simulink model "htx_ekf_base"  (R2024b)
settings: Solver=FixedStepAuto  StartTime=0.0  StopTime=10.0  RelTol=1e-3
undefined symbols (not defined in the file): chi, GR, params, rpm2rad_s, segment_data
libraries: simulink_extras x4, matrix_library x1
settings Model: Creator=lukec  LastModifiedBy=lukec
settings OptimizationCC: DefaultParameterBehavior=Inlined  EnhancedBackFolding=on  PassReuseOutputArgsAs=Individual arguments  ZeroExternalMemoryAtStartup=off  ZeroInternalMemoryAtStartup=off  OptimizeBlockOrder=speed  DifferentSizesBufferReuse=on  OptimizationCustomize=off  EfficientTunableParamExpr=on
settings DebuggingCC: ParameterTunabilityLossMsg=error
settings HardwareCC: ProdBitPerPointer=32  ProdBitPerSizeT=32  ProdBitPerPtrDiffT=32  ProdLargestAtomicInteger=Long  ProdLargestAtomicFloat=Double  ProdWordSize=32  ProdHWDeviceType=ARM Compatible->ARM Cortex-M
settings SFSimCC: MATLABDynamicMemAlloc=off
settings RTWCC: Description=Embedded Coder  SystemTargetFile=ert.tlc  GenCodeOnly=on  PackageGeneratedCodeAndArtifacts=on  TemplateMakefile=ert_default_tmf  Toolchain=CMake  TargetLang=C++
settings CodeAppCC: ForceParamTrailComments=on  IgnoreCustomStorageClasses=off  MaxIdLength=255  OperatorAnnotations=on  SimulinkDataObjDesc=on  SFDataObjDesc=on  InsertBlockDesc=on
settings ERTTargetCC: TargetLangStandard=C++17 (ISO)  CodeInterfacePackaging=C++ class  RootIOFormat=Structure reference  ERTCustomFileTemplate=example_file_process.tlc  ArrayContainerType=std::array

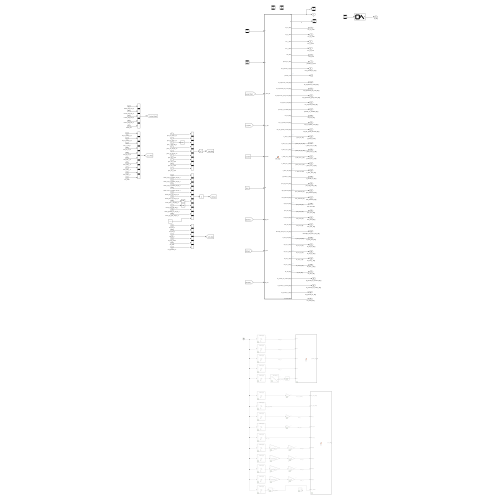
[thumbnail: Simulink's stored preview of the top-level diagram]
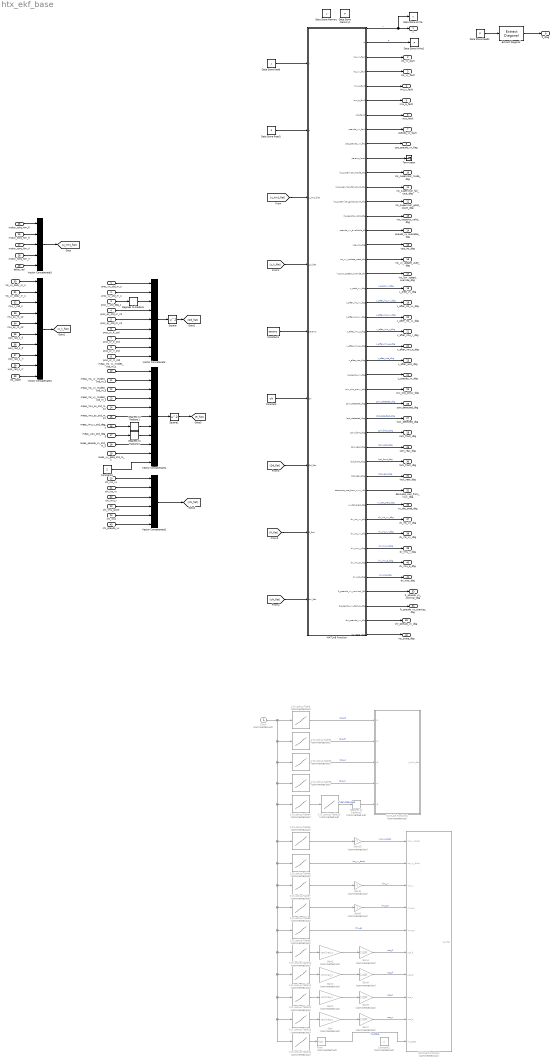
== system htx_ekf_base ==
  proc_vx_std_m_s : Inport
  proc_vy_std_m_s : Inport  Port=2
  proc_r_std_deg_s : Inport  Port=3
  proc_ax_std_m_s2 : Inport  Port=4
  proc_ay_std_m_s2 : Inport  Port=5
  proc_sr_fl_std : Inport  Port=6
  proc_sr_fr_std : Inport  Port=7
  proc_sr_rl_std : Inport  Port=8
  proc_sr_rr_std : Inport  Port=9
  meas_ins_vx_mode1_std_m_s : Inport  Port=10
  meas_ins_vy_mode1_std_m_s : Inport  Port=11
  meas_ins_vx_mode2_std_m_s : Inport  Port=12
  meas_ins_vy_mode2_std_m_s : Inport  Port=13
  meas_imu_ax_std_m_s2 : Inport  Port=14
  meas_imu_ay_std_m_s2 : Inport  Port=15
  meas_imu_r_std_deg_s : Inport  Port=16
  meas_wss_std_deg_s : Inport  Port=17
  meas_pseudo_vx_std_m_s : Inport  Port=18
  meas_vy_gate_std_m_s : Inport  Port=19
  chi_ins_vx : Inport  Port=20
  chi_ins_vy : Inport  Port=21
  chi_imu_r : Inport  Port=22
  chi_imu_accel : Inport  Port=23
  chi_wss : Inport  Port=24
  motor_torq_Nm_fl : Inport  Port=25
  motor_torq_Nm_fr : Inport  Port=26
  motor_torq_Nm_rl : Inport  Port=27
  motor_torq_Nm_rr : Inport  Port=28
  delta_rad : Inport  Port=29
  ins_vx_body_m_s : Inport  Port=30
  ins_vy_body_m_s : Inport  Port=31
  imu_r_rad_s : Inport  Port=32
  imu_ax_m_s2 : Inport  Port=33
  imu_ay_m_s2 : Inport  Port=34
  wss_rad_s_fl : Inport  Port=35
  wss_rad_s_fr : Inport  Port=36
  wss_rad_s_rl : Inport  Port=37
  wss_rad_s_rr : Inport  Port=38
  ins_state : Inport  Port=39
  chi_pseudo_vx : Inport  Port=40
  1-D Lookup Table : Lookup_n-D  Commented=on  NumberOfTableDimensions=1  BreakpointsForDimension1=segment_data.globalTime  Table=segment_data.inv1_dynamics.actual_torque_nm  ExtrapMethod=Clip  InternalRulePriority=Speed  RndMeth=Simplest
  1-D Lookup Table1 : Lookup_n-D  Commented=on  NumberOfTableDimensions=1  BreakpointsForDimension1=segment_data.globalTime  Table=segment_data.inv2_dynamics.actual_torque_nm  ExtrapMethod=Clip  InternalRulePriority=Speed  RndMeth=Simplest
  1-D Lookup Table10 : Lookup_n-D  Commented=on  NumberOfTableDimensions=1  BreakpointsForDimension1=segment_data.globalTime  Table=segment_data.inv1_dynamics.actual_speed_rpm  ExtrapMethod=Clip  InternalRulePriority=Speed  RndMeth=Simplest
  1-D Lookup Table11 : Lookup_n-D  Commented=on  NumberOfTableDimensions=1  BreakpointsForDimension1=segment_data.globalTime  Table=segment_data.inv2_dynamics.actual_speed_rpm  ExtrapMethod=Clip  InternalRulePriority=Speed  RndMeth=Simplest
  1-D Lookup Table12 : Lookup_n-D  Commented=on  NumberOfTableDimensions=1  BreakpointsForDimension1=segment_data.globalTime  Table=segment_data.inv3_dynamics.actual_speed_rpm  ExtrapMethod=Clip  InternalRulePriority=Speed  RndMeth=Simplest
  1-D Lookup Table13 : Lookup_n-D  Commented=on  NumberOfTableDimensions=1  BreakpointsForDimension1=segment_data.globalTime  Table=segment_data.inv4_dynamics.actual_speed_rpm  ExtrapMethod=Clip  InternalRulePriority=Speed  RndMeth=Simplest
  1-D Lookup Table14 : Lookup_n-D  Commented=on  NumberOfTableDimensions=1  BreakpointsForDimension1=segment_data.globalTime  Table=segment_data.VNData.status.ins_mode_int  ExtrapMethod=Clip  InternalRulePriority=Speed  RndMeth=Simplest
  1-D Lookup Table15 : Lookup_n-D  Commented=on  NumberOfTableDimensions=1  BreakpointsForDimension1=[1060 3010]  Table=[23 -23]  ExtrapMethod=Clip  InternalRulePriority=Speed  RndMeth=Simplest
  1-D Lookup Table2 : Lookup_n-D  Commented=on  NumberOfTableDimensions=1  BreakpointsForDimension1=segment_data.globalTime  Table=segment_data.inv3_dynamics.actual_torque_nm  ExtrapMethod=Clip  InternalRulePriority=Speed  RndMeth=Simplest
  1-D Lookup Table3 : Lookup_n-D  Commented=on  NumberOfTableDimensions=1  BreakpointsForDimension1=segment_data.globalTime  Table=segment_data.inv4_dynamics.actual_torque_nm  ExtrapMethod=Clip  InternalRulePriority=Speed  RndMeth=Simplest
  1-D Lookup Table4 : Lookup_n-D  Commented=on  NumberOfTableDimensions=1  BreakpointsForDimension1=segment_data.globalTime  Table=segment_data.steering_data.steering_analog_raw  ExtrapMethod=Clip  InternalRulePriority=Speed  RndMeth=Simplest
  1-D Lookup Table5 : Lookup_n-D  Commented=on  NumberOfTableDimensions=1  BreakpointsForDimension1=segment_data.globalTime  Table=segment_data.VNData.vn_vel_m_s.x  ExtrapMethod=Clip  InternalRulePriority=Speed  RndMeth=Simplest
  1-D Lookup Table6 : Lookup_n-D  Commented=on  NumberOfTableDimensions=1  BreakpointsForDimension1=segment_data.globalTime  Table=segment_data.VNData.vn_vel_m_s.y  ExtrapMethod=Clip  InternalRulePriority=Speed  RndMeth=Simplest
  1-D Lookup Table7 : Lookup_n-D  Commented=on  NumberOfTableDimensions=1  BreakpointsForDimension1=segment_data.globalTime  Table=segment_data.VNData.vn_angular_rate_rad_s.z  ExtrapMethod=Clip  InternalRulePriority=Speed  RndMeth=Simplest
  1-D Lookup Table8 : Lookup_n-D  Commented=on  NumberOfTableDimensions=1  BreakpointsForDimension1=segment_data.globalTime  Table=segment_data.VNData.vn_linear_accel_m_ss.x  ExtrapMethod=Clip  InternalRulePriority=Speed  RndMeth=Simplest
  1-D Lookup Table9 : Lookup_n-D  Commented=on  NumberOfTableDimensions=1  BreakpointsForDimension1=segment_data.globalTime  Table=segment_data.VNData.vn_linear_accel_m_ss.y  ExtrapMethod=Clip  InternalRulePriority=Speed  RndMeth=Simplest
  Clock : Clock  Commented=on
  Constant : Constant  Value=chi  OutDataTypeStr=Bus: chi_bus
  Constant1 : Constant  Value=params  OutDataTypeStr=Bus: params_bus
  Constant2 : Constant  Commented=on  Value=0
  Constant3 : Constant  Value=2
  Data Store Memory : DataStoreMemory  DataStoreName=x  WriteAfterWriteMsg=warning  InitialValue=x0  ShowAdditionalParam=off
  Data Store Memory1 : DataStoreMemory  DataStoreName=P  WriteAfterWriteMsg=warning  InitialValue=P0  ShowAdditionalParam=off
  Data Store Read : DataStoreRead  DataStoreName=x  IndexOptions=Index vector (dialog)  Indices=1  OutputSizes=1
  Data Store Read1 : DataStoreRead  DataStoreName=P  IndexOptions=Index vector (dialog)  Indices=1  OutputSizes=1
  Data Store Read2 : DataStoreRead  DataStoreName=P  IndexOptions=Index vector (dialog)  Indices=1  OutputSizes=1
  Data Store Write : DataStoreWrite  DataStoreName=x  IndexOptions=Index vector (dialog)  Indices=1  OutputSizes=1
  Data Store Write1 : DataStoreWrite  DataStoreName=P  IndexOptions=Index vector (dialog)  Indices=1  OutputSizes=1
  Degrees to Radians : simulink_extras/Transformations/Degrees to Radians
  Degrees to Radians1 : simulink_extras/Transformations/Degrees to Radians
  Degrees to Radians2 : simulink_extras/Transformations/Degrees to Radians
  Degrees to Radians3 : simulink_extras/Transformations/Degrees to Radians  Commented=on
  Extract Diagonal : matrix_library/Extract Diagonal
      settings: LibrarySourceBlock=|
      | simulink/Matrix
      | Operations/Extract Diagonal
  Floor : Rounding  Commented=on
  Gain{,1..3} (4 alike) : Gain  Commented=on  Gain=rpm2rad_s
  Gain10 : Gain  Commented=on  Gain=-1
  Gain{4..7} (4 alike) : Gain  Commented=on  Gain=1/GR
  Gain8 : Gain  Commented=on  Gain=-1
  Gain9 : Gain  Commented=on  Gain=-1
  MATLAB Function : MATLAB Function  TreatAsAtomicUnit=on
  MATLAB Function1 : MATLAB Function  Commented=on  TreatAsAtomicUnit=on
  MATLAB Function2 : MATLAB Function  Commented=on  TreatAsAtomicUnit=on
  Square : Math  Operator=square
  Square1 : Math  Operator=square
  Terminator : Terminator
  Vector Concatenate : Concatenate  NumInputs=9
  Vector Concatenate1 : Concatenate  NumInputs=11
  Vector Concatenate2 : Concatenate  NumInputs=6
  Vector Concatenate3 : Concatenate  NumInputs=5
  Vector Concatenate4 : Concatenate  NumInputs=10
  x : Outport
  ins_vx_fault : Outport  Port=2
  ins_vy_fault : Outport  Port=3
  imu_r_fault : Outport  Port=4
  imu_a_fault : Outport  Port=5
  wss_fault : Outport  Port=6
  pseudo_vx_fault : Outport  Port=7
  use_pseudo_vx_flag : Outport  Port=8
  P_diag : Outport  Port=9
  ins_supervisor_mode_dbg : Outport  Port=10
  ins_supervisor_fail_cout_dbg : Outport  Port=11
  ins_supervisor_good_count_dbg : Outport  Port=12
  ins_resports_valid_dbg : Outport  Port=13
  pseudo_vx_available_dbg : Outport  Port=14
  use_ins_dbg : Outport  Port=15
  ins_vx_update_used_dbg : Outport  Port=16
  ins_low_speed_override_dbg : Outport  Port=17
  x_pred_vx_dbg : Outport  Port=18
  x_after_ins_vx_dbg : Outport  Port=19
  x_after_ins_vy_dbg : Outport  Port=20
  x_after_imu_r_dbg : Outport  Port=21
  x_after_imu_a_dbg : Outport  Port=22
  x_after_wss_dbg : Outport  Port=23
  z_pseudo_vx_dbg : Outport  Port=24
  pvx_slip_proxy_dbg : Outport  Port=25
  spin_detected_dbg : Outport  Port=26
  lock_detected_dbg : Outport  Port=27
  spin_front_dbg : Outport  Port=28
  spin_rear_dbg : Outport  Port=29
  lock_front_dbg : Outport  Port=30
  lock_rear_dbg : Outport  Port=31
  decouple_wss_from_vxvy_dbg : Outport  Port=32
  R_pseudo_vx_nominal_dbg : Outport  Port=33
  R_pseudo_vx_startup_dbg : Outport  Port=34
  chi_pseudo_vx_dbg : Outport  Port=35
  vx_dot_pred_dbg : Outport  Port=36
  dv_ins_vx_dbg : Outport  Port=37
  dv_ins_vy_dbg : Outport  Port=38
  dv_imu_r_dbg : Outport  Port=39
  dv_imu_a_dbg : Outport  Port=40
  dv_wss_dbg : Outport  Port=41
  ins_state_dbg : Outport  Port=42
  wires:
  Data Store Read/1 -> MATLAB Function/1("x ")
  Data Store Read1/1 -> MATLAB Function/2("P ")
  Constant1/1 -> MATLAB Function/5(params)
  Constant/1 -> MATLAB Function/6(chi)
  MATLAB Function/1(x) -> Data Store Write/1, x/1  "x"
  MATLAB Function/2(P) -> Data Store Write1/1  "P"
  Clock/1 -> 1-D Lookup Table4/1, 1-D Lookup Table5/1, 1-D Lookup Table13/1, 1-D Lookup Table14/1, 1-D Lookup Table12/1, 1-D Lookup Table11/1, 1-D Lookup Table10/1, 1-D Lookup Table9/1, 1-D Lookup Table8/1, 1-D Lookup Table7/1, 1-D Lookup Table6/1, 1-D Lookup Table3/1, 1-D Lookup Table2/1, 1-D Lookup Table1/1, 1-D Lookup Table/1
  1-D Lookup Table/1 -> MATLAB Function1/1(u1)  "torq_fl"
  1-D Lookup Table1/1 -> MATLAB Function1/2(u2)  "torq_fr"
  1-D Lookup Table2/1 -> MATLAB Function1/3(u3)  "torq_rl"
  1-D Lookup Table3/1 -> MATLAB Function1/4(u4)  "torq_rr"
  1-D Lookup Table4/1 -> 1-D Lookup Table15/1
  1-D Lookup Table7/1 -> Gain9/1
  1-D Lookup Table8/1 -> Gain8/1
  1-D Lookup Table9/1 -> MATLAB Function2/5(imu_ay)  "imu_ay"
  1-D Lookup Table10/1 -> Gain3/1
  1-D Lookup Table11/1 -> Gain2/1
  1-D Lookup Table12/1 -> Gain1/1
  1-D Lookup Table13/1 -> Gain/1
  [u_km1_flat] -> MATLAB Function/3(u_km1_flat)
  [z_k_flat] -> MATLAB Function/4(z_k_flat)
  MATLAB Function/3(ins_vx_fault) -> ins_vx_fault/1
  MATLAB Function/4(ins_vy_fault) -> ins_vy_fault/1
  MATLAB Function/5(imu_r_fault) -> imu_r_fault/1
  MATLAB Function/6(imu_a_fault) -> imu_a_fault/1
  MATLAB Function/7(wss_fault) -> wss_fault/1
  MATLAB Function/8(pseudo_vx_fault) -> pseudo_vx_fault/1
  MATLAB Function/9(use_pseudo_vx_flag) -> use_pseudo_vx_flag/1
  Data Store Read2/1 -> Extract Diagonal/1
  Extract Diagonal/1 -> P_diag/1
  proc_vx_std_m_s/1 -> Vector Concatenate/1
  proc_vy_std_m_s/1 -> Vector Concatenate/2
  proc_r_std_deg_s/1 -> Degrees to Radians/1
  proc_ax_std_m_s2/1 -> Vector Concatenate/4
  proc_ay_std_m_s2/1 -> Vector Concatenate/5
  proc_sr_fl_std/1 -> Vector Concatenate/6
  proc_sr_fr_std/1 -> Vector Concatenate/7
  proc_sr_rl_std/1 -> Vector Concatenate/8
  proc_sr_rr_std/1 -> Vector Concatenate/9
  Degrees to Radians/1 -> Vector Concatenate/3
  Vector Concatenate/1 -> Square/1
  Square/1 -> [Qd_flat]
  [Qd_flat] -> MATLAB Function/7(Qd_flat)
  meas_imu_r_std_deg_s/1 -> Degrees to Radians1/1
  meas_wss_std_deg_s/1 -> Degrees to Radians2/1
  Degrees to Radians1/1 -> Vector Concatenate1/7
  Degrees to Radians2/1 -> Vector Concatenate1/8
  meas_pseudo_vx_std_m_s/1 -> Vector Concatenate1/9
  meas_vy_gate_std_m_s/1 -> Vector Concatenate1/10
  meas_imu_ay_std_m_s2/1 -> Vector Concatenate1/6
  meas_imu_ax_std_m_s2/1 -> Vector Concatenate1/5
  meas_ins_vy_mode1_std_m_s/1 -> Vector Concatenate1/2
  meas_ins_vx_mode1_std_m_s/1 -> Vector Concatenate1/1
  Vector Concatenate1/1 -> Square1/1
  Square1/1 -> [R_flat]
  [R_flat] -> MATLAB Function/8(R_flat)
  chi_ins_vx/1 -> Vector Concatenate2/1
  chi_ins_vy/1 -> Vector Concatenate2/2
  chi_imu_r/1 -> Vector Concatenate2/3
  chi_imu_accel/1 -> Vector Concatenate2/4
  chi_wss/1 -> Vector Concatenate2/5
  Vector Concatenate2/1 -> [chi_flat]
  [chi_flat] -> MATLAB Function/9(chi_flat)
  motor_torq_Nm_fl/1 -> Vector Concatenate3/1
  motor_torq_Nm_fr/1 -> Vector Concatenate3/2
  motor_torq_Nm_rl/1 -> Vector Concatenate3/3
  motor_torq_Nm_rr/1 -> Vector Concatenate3/4
  delta_rad/1 -> Vector Concatenate3/5
  ins_vx_body_m_s/1 -> Vector Concatenate4/1
  ins_vy_body_m_s/1 -> Vector Concatenate4/2
  wss_rad_s_fl/1 -> Vector Concatenate4/6
  wss_rad_s_fr/1 -> Vector Concatenate4/7
  wss_rad_s_rl/1 -> Vector Concatenate4/8
  wss_rad_s_rr/1 -> Vector Concatenate4/9
  ins_state/1 -> Vector Concatenate4/10
  imu_ay_m_s2/1 -> Vector Concatenate4/5
  imu_ax_m_s2/1 -> Vector Concatenate4/4
  imu_r_rad_s/1 -> Vector Concatenate4/3
  MATLAB Function/10(params_local) -> Terminator/1
  meas_ins_vx_mode2_std_m_s/1 -> Vector Concatenate1/3
  meas_ins_vy_mode2_std_m_s/1 -> Vector Concatenate1/4
  MATLAB Function/11(ins_supervisor_mode_dbg) -> ins_supervisor_mode_dbg/1
  MATLAB Function/12(ins_supervisor_fail_count_dbg) -> ins_supervisor_fail_cout_dbg/1
  MATLAB Function/13(ins_supervisor_good_count_dbg) -> ins_supervisor_good_count_dbg/1
  MATLAB Function/14(ins_reports_valid_dbg) -> ins_resports_valid_dbg/1
  MATLAB Function/15(pseudo_vx_available_dbg) -> pseudo_vx_available_dbg/1
  MATLAB Function/16(use_ins_dbg) -> use_ins_dbg/1
  MATLAB Function/17(ins_vx_update_used_dbg) -> ins_vx_update_used_dbg/1
  MATLAB Function/18(ins_low_speed_override_dbg) -> ins_low_speed_override_dbg/1
  1-D Lookup Table14/1 -> Floor/1
  1-D Lookup Table15/1 -> Degrees to Radians3/1  "wheel_steer_deg"
  Gain/1 -> Gain7/1
  Gain1/1 -> Gain6/1
  Gain2/1 -> Gain5/1
  Gain3/1 -> Gain4/1
  Gain4/1 -> MATLAB Function2/6(wss_fl)  "wss_fl"
  Gain5/1 -> MATLAB Function2/7(wss_fr)  "wss_fr"
  Gain6/1 -> MATLAB Function2/8(wss_rl)  "wss_rl"
  Gain7/1 -> MATLAB Function2/9(wss_rr)  "wss_rr"
  Gain8/1 -> MATLAB Function2/4(imu_ax)  "imu_ax"
  Gain9/1 -> MATLAB Function2/3(imu_r)  "imu_r"
  Degrees to Radians3/1 -> MATLAB Function1/5(u5)
  1-D Lookup Table5/1 -> Gain10/1
  Gain10/1 -> MATLAB Function2/1(ins_vx_body)  "ins_vx_body"
  1-D Lookup Table6/1 -> MATLAB Function2/2(ins_vy_body)  "ins_vy_body"
  Floor/1 -> MATLAB Function2/10(ins_state)  "ins_state"
  Vector Concatenate3/1 -> [u_km1_flat]
  Vector Concatenate4/1 -> [z_k_flat]
  Constant3/1 -> Vector Concatenate1/11
  chi_pseudo_vx/1 -> Vector Concatenate2/6
  MATLAB Function/19(x_pred_vx_dbg) -> x_pred_vx_dbg/1  "x_pred_vx_dbg"
  MATLAB Function/20(x_after_ins_vx_dbg) -> x_after_ins_vx_dbg/1  "x_after_ins_vx_dbg"
  MATLAB Function/21(x_after_ins_vy_dbg) -> x_after_ins_vy_dbg/1  "x_after_ins_vy_dbg"
  MATLAB Function/22(x_after_imu_r_dbg) -> x_after_imu_r_dbg/1  "x_after_imu_r_dbg"
  MATLAB Function/23(x_after_imu_a_dbg) -> x_after_imu_a_dbg/1  "x_after_imu_a_dbg"
  MATLAB Function/24(x_after_wss_dbg) -> x_after_wss_dbg/1  "x_after_wss_dbg"
  MATLAB Function/25(z_pseudo_vx_dbg) -> z_pseudo_vx_dbg/1
  MATLAB Function/26(pvx_slip_proxy_dbg) -> pvx_slip_proxy_dbg/1
  MATLAB Function/27(spin_detected_dbg) -> spin_detected_dbg/1  "spin_detected_dbg"
  MATLAB Function/28(lock_detected_dbg) -> lock_detected_dbg/1  "lock_detected_dbg"
  MATLAB Function/29(spin_front_dbg) -> spin_front_dbg/1  "spin_front_dbg"
  MATLAB Function/30(spin_rear_dbg) -> spin_rear_dbg/1  "spin_rear_dbg"
  MATLAB Function/31(lock_front_dbg) -> lock_front_dbg/1  "lock_front_dbg"
  MATLAB Function/32(lock_rear_dbg) -> lock_rear_dbg/1  "lock_rear_dbg"
  MATLAB Function/33(decouple_wss_from_vxvy_dbg) -> decouple_wss_from_vxvy_dbg/1
  MATLAB Function/40(R_pseudo_vx_nominal_dbg) -> R_pseudo_vx_nominal_dbg/1
  MATLAB Function/41(R_pseudo_vx_startup_dbg) -> R_pseudo_vx_startup_dbg/1
  MATLAB Function/42(chi_pseudo_vx_dbg) -> chi_pseudo_vx_dbg/1
  MATLAB Function/34(vx_dot_pred_dbg) -> vx_dot_pred_dbg/1  "vx_dot_pred_dbg"
  MATLAB Function/35(dv_ins_vx_dbg) -> dv_ins_vx_dbg/1  "dv_ins_vx_dbg"
  MATLAB Function/36(dv_ins_vy_dbg) -> dv_ins_vy_dbg/1  "dv_ins_vy_dbg"
  MATLAB Function/37(dv_imu_r_dbg) -> dv_imu_r_dbg/1  "dv_imu_r_dbg"
  MATLAB Function/38(dv_imu_a_dbg) -> dv_imu_a_dbg/1  "dv_imu_a_dbg"
  MATLAB Function/39(dv_wss_dbg) -> dv_wss_dbg/1  "dv_wss_dbg"
  MATLAB Function/43(ins_state_dbg) -> ins_state_dbg/1

== matlab function htx_ekf_base/MATLAB Function2 ==
  data: ins_vx_body input; z_k_flat output; ins_vy_body input; imu_r input; imu_ax input; imu_ay input; wss_fl input; wss_fr input; wss_rl input; wss_rr input; ins_state input
function z_k_flat = fcn(ins_vx_body, ins_vy_body, imu_r, imu_ax, imu_ay, wss_fl, wss_fr, wss_rl, wss_rr, ins_state)
    z_k_flat = [ins_vx_body;
                ins_vy_body;
                imu_r;
                imu_ax;
                imu_ay;
                wss_fl;
                wss_fr;
                wss_rl;
                wss_rr;
                ins_state];

== matlab function htx_ekf_base/MATLAB Function1 ==
  data: u1 input; u_km1_flat output; u2 input; u3 input; u4 input; u5 input
function u_km1_flat = fcn(u1, u2, u3, u4, u5)
    u_km1_flat = [u1; u2; u3; u4; u5];

== matlab function htx_ekf_base/MATLAB Function ==
  data: x input; x output; P input; u_km1_flat input; z_k_flat input; params input; chi input; P output; ins_vx_fault output; ins_vy_fault output; imu_r_fault output; imu_a_fault output; wss_fault output; pseudo_vx_fault output; use_pseudo_vx_flag output; Qd_flat input; R_flat input; chi_flat input; params_local output Bus: params_bus; ins_supervisor_mode_dbg output; ins_supervisor_fail_count_dbg output; ins_supervisor_good_count_dbg output; ins_reports_valid_dbg output; pseudo_vx_available_dbg output; use_ins_dbg output; ins_vx_update_used_dbg output; ins_low_speed_override_dbg output; x_pred_vx_dbg output; x_after_ins_vx_dbg output; x_after_ins_vy_dbg output; x_after_imu_r_dbg output; x_after_imu_a_dbg output; x_after_wss_dbg output; z_pseudo_vx_dbg output; pvx_slip_proxy_dbg output; spin_detected_dbg output; lock_detected_dbg output; spin_front_dbg output; spin_rear_dbg output; lock_front_dbg output; lock_rear_dbg output; decouple_wss_from_vxvy_dbg output; vx_dot_pred_dbg output; dv_ins_vx_dbg output; dv_ins_vy_dbg output; dv_imu_r_dbg output; dv_imu_a_dbg output; dv_wss_dbg output; R_pseudo_vx_nominal_dbg output; R_pseudo_vx_startup_dbg output; chi_pseudo_vx_dbg output; ins_state_dbg output
function [x, P, ...
    ins_vx_fault, ins_vy_fault, imu_r_fault, imu_a_fault, wss_fault, pseudo_vx_fault, ...
    use_pseudo_vx_flag, params_local, ...
    ins_supervisor_mode_dbg, ins_supervisor_fail_count_dbg, ins_supervisor_good_count_dbg, ...
    ins_reports_valid_dbg, pseudo_vx_available_dbg, use_ins_dbg, ...
    ins_vx_update_used_dbg, ins_low_speed_override_dbg, ...
    x_pred_vx_dbg, x_after_ins_vx_dbg, x_after_ins_vy_dbg, x_after_imu_r_dbg, ...
    x_after_imu_a_dbg, x_after_wss_dbg, z_pseudo_vx_dbg, pvx_slip_proxy_dbg, ...
    spin_detected_dbg, lock_detected_dbg, spin_front_dbg, spin_rear_dbg, ...
    lock_front_dbg, lock_rear_dbg, decouple_wss_from_vxvy_dbg, ...
    vx_dot_pred_dbg, dv_ins_vx_dbg, dv_ins_vy_dbg, dv_imu_r_dbg, dv_imu_a_dbg, dv_wss_dbg, ...
    R_pseudo_vx_nominal_dbg, R_pseudo_vx_startup_dbg, chi_pseudo_vx_dbg, ins_state_dbg] = ...
    ekf_step(x, P, u_km1_flat, z_k_flat, params, chi, Qd_flat, R_flat, chi_flat)

    %--------------------------------------------------------------
    % Unpack inputs, thx simulink
    %--------------------------------------------------------------
    u_km1.motor_torq_fl = u_km1_flat(1);
    u_km1.motor_torq_fr = u_km1_flat(2);
    u_km1.motor_torq_rl = u_km1_flat(3);
    u_km1.motor_torq_rr = u_km1_flat(4);
    u_km1.delta         = u_km1_flat(5);

    z_k.ins_vx_body = z_k_flat(1);
    z_k.ins_vy_body = z_k_flat(2);
    z_k.imu_r       = z_k_flat(3);
    z_k.imu_ax      = z_k_flat(4);
    z_k.imu_ay      = z_k_flat(5);
    z_k.wss_fl      = z_k_flat(6);
    z_k.wss_fr      = z_k_flat(7);
    z_k.wss_rl      = z_k_flat(8);
    z_k.wss_rr      = z_k_flat(9);
    z_k.ins_state   = z_k_flat(10);

    %--------------------------------------------------------------
    % Params unpacking, thx simulink
    %--------------------------------------------------------------
    params.decouple_wss_from_vxvy = false;

    params.Qd_base = diag(Qd_flat);
    params.Qd      = params.Qd_base;

    params.R_ins_vel       = diag([0, 0]); % placeholder, if mode 0, INS is rejected
    params.R_ins_vel_mode1 = diag([R_flat(1), R_flat(2)]);
    params.R_ins_vel_mode2 = diag([R_flat(3), R_flat(4)]);
    params.R_imu_a         = diag([R_flat(5), R_flat(6)]);
    params.R_imu_r         = R_flat(7);
    params.R_wss           = R_flat(8) * eye(4);

    params.R_pseudo_vx         = R_flat(9);
    params.R_pseudo_vx_nominal = R_flat(9);
    params.R_vy_gate           = R_flat(10);

    if numel(R_flat) >= 11
        params.R_pseudo_vx_startup = R_flat(11);
    else
        params.R_pseudo_vx_startup = 4.0;
    end

    %--------------------------------------------------------------
    % Chi probabilities
    %--------------------------------------------------------------
    chi.ins_vx    = chi_flat(1);
    chi.ins_vy    = chi_flat(2);
    chi.imu_r     = chi_flat(3);
    chi.imu_accel = chi_flat(4);
    chi.wss       = chi_flat(5);

    if numel(chi_flat) >= 6
        chi.pseudo_vx = chi_flat(6);
    else
        chi.pseudo_vx = chi.ins_vx;
    end

    %--------------------------------------------------------------
    % Run EKF
    %--------------------------------------------------------------
    [x, P, flags, ~, use_pseudo_vx, params_local, ...
        ins_supervisor_mode_dbg, ins_supervisor_fail_count_dbg, ins_supervisor_good_count_dbg, ...
        ins_reports_valid_dbg, pseudo_vx_available_dbg, use_ins_dbg, ...
        ins_vx_update_used_dbg, ins_low_speed_override_dbg, ...
        x_pred_vx_dbg, x_after_ins_vx_dbg, x_after_ins_vy_dbg, x_after_imu_r_dbg, ...
        x_after_imu_a_dbg, x_after_wss_dbg, z_pseudo_vx_dbg, pvx_slip_proxy_dbg, ...
        spin_detected_dbg, lock_detected_dbg, spin_front_dbg, spin_rear_dbg, ...
        lock_front_dbg, lock_rear_dbg, decouple_wss_from_vxvy_dbg, ...
        vx_dot_pred_dbg, dv_ins_vx_dbg, dv_ins_vy_dbg, dv_imu_r_dbg, dv_imu_a_dbg, dv_wss_dbg, ins_state_dbg] = ...
        vxvy_sr_ekf_step(x, P, u_km1, z_k, params, chi);

    %--------------------------------------------------------------
    % Fault outputs
    %--------------------------------------------------------------
    ins_vx_fault    = flags.ins_vx;
    ins_vy_fault    = flags.ins_vy;
    imu_r_fault     = flags.imu_r;
    imu_a_fault     = flags.imu_a;
    wss_fault       = flags.wss;
    pseudo_vx_fault = flags.pseudo_vx;

    use_pseudo_vx_flag = use_pseudo_vx;

    %--------------------------------------------------------------
    % passthrough debug params
    %--------------------------------------------------------------
    R_pseudo_vx_nominal_dbg = params.R_pseudo_vx_nominal;
    R_pseudo_vx_startup_dbg = params.R_pseudo_vx_startup;
    chi_pseudo_vx_dbg       = chi.pseudo_vx;
end
